simulink model "BDA_DynamicModel_v3"  (R2021b)
settings: Solver=ode23t  StartTime=0.0  StopTime=15  FixedStep=0.000001  MaxStep=1e-5  MinStep=1e-7  RelTol=1e-3
undefined symbols (not defined in the file or in its folder): X, Y, Z
libraries: sm_lib x47, nesl_utility x7
(part 1 of 5)
settings Model: Creator=Alejandro TeveraRuiz  LastModifiedBy=Alejandro TeveraRuiz

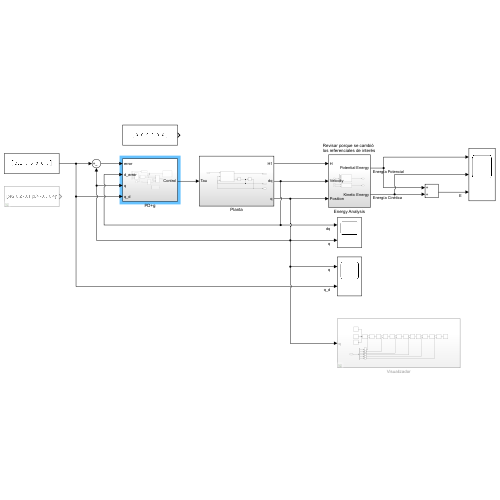
[thumbnail: Simulink's stored preview of the top-level diagram]
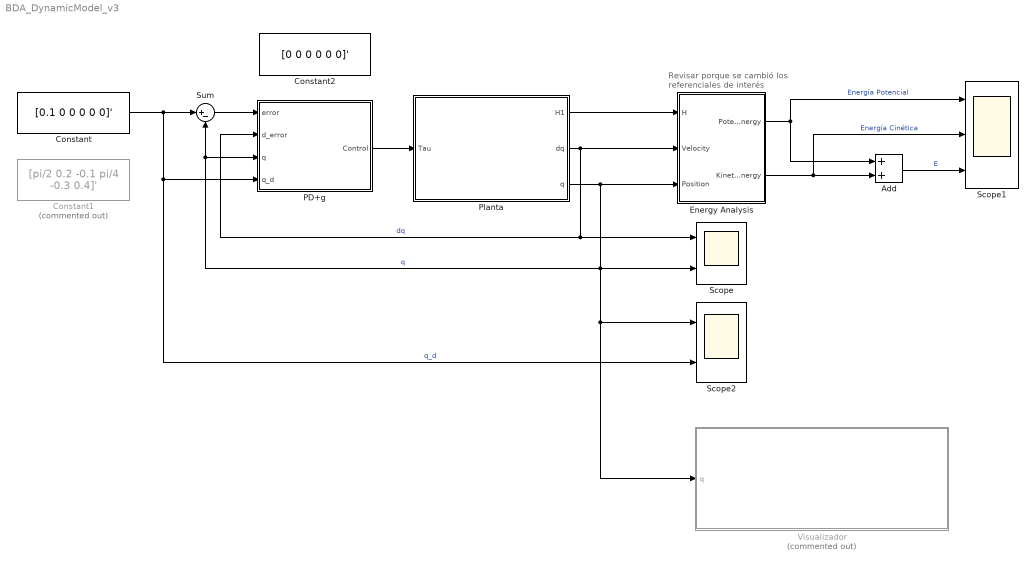
== system BDA_DynamicModel_v3 ==
  note: Revisar porque se cambió los referenciales de interés
  Add : Sum
  Constant : Constant  Value=[0.1 0 0 0 0 0]'
  Constant1 : Constant  Commented=on  Value=[pi/2 0.2 -0.1 pi/4 -0.3 0.4]'
  Constant2 : Constant  Value=[0 0 0 0 0 0]'
  Energy Analysis : Subsystem
  PD+g : Subsystem
  Planta : Subsystem
  Scope : Scope  NumInputPorts=2
  Scope1 : Scope  NumInputPorts=3
  Scope2 : Scope  NumInputPorts=2
  Sum : Sum  Inputs=|+-
  Visualizador : Subsystem  Commented=on
  wires:
  Energy Analysis/1(Potential Energy) -> Scope1/1, Add/1  "Energía Potencial"
  Energy Analysis/2(Kinetic Energy) -> Add/2, Scope1/2  "Energía Cinética"
  Constant/1 -> PD+g/4(q_d), Scope2/2, Sum/1  "q_d"
  Sum/1 -> PD+g/1(error)
  Planta/1(H1) -> Energy Analysis/1(H)
  Planta/2(dq) -> PD+g/2(d_error), Scope/1, Energy Analysis/2(Velocity)  "dq"
  Planta/3(q) -> Energy Analysis/3(Position), Visualizador/1(q), Scope2/1, PD+g/3(q), Sum/2, Scope/2  "q"
  Add/1 -> Scope1/3  "E"
  PD+g/1(Control) -> Planta/1(Tau)

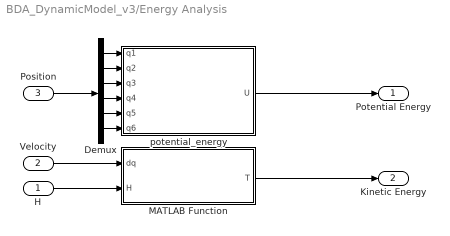
== system BDA_DynamicModel_v3/Energy Analysis ==
  H : Inport
  Velocity : Inport  Port=2
  Position : Inport  Port=3
  Demux : Demux  Outputs=6
  MATLAB Function : MATLAB Function  TreatAsAtomicUnit=on
  potential_energy : MATLAB Function  TreatAsAtomicUnit=on
  Potential Energy : Outport
  Kinetic Energy : Outport  Port=2
  wires:
  Demux/3 -> potential_energy/3(q3)
  Velocity/1 -> MATLAB Function/1(dq)
  Demux/5 -> potential_energy/5(q5)
  Demux/4 -> potential_energy/4(q4)
  Demux/2 -> potential_energy/2(q2)
  Demux/1 -> potential_energy/1(q1)
  Demux/6 -> potential_energy/6(q6)
  H/1 -> MATLAB Function/2(H)
  MATLAB Function/1(T) -> Kinetic Energy/1
  Position/1 -> Demux/1
  potential_energy/1(U) -> Potential Energy/1

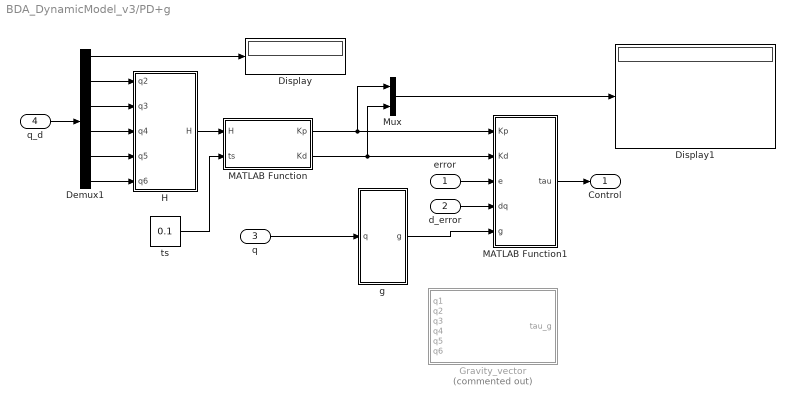
== system BDA_DynamicModel_v3/PD+g ==
  error : Inport
  d_error : Inport  Port=2
  q : Inport  Port=3  PortDimensions=[6,1]
  q_d : Inport  Port=4
  Demux1 : Demux  Outputs=6
  Display : Display
  Display1 : Display
  Gravity_vector : MATLAB Function  Commented=on  TreatAsAtomicUnit=on
  H : MATLAB Function  TreatAsAtomicUnit=on
  MATLAB Function : MATLAB Function  TreatAsAtomicUnit=on
  MATLAB Function1 : MATLAB Function  TreatAsAtomicUnit=on
  Mux : Mux  Inputs=2
  g : MATLAB Function  TreatAsAtomicUnit=on
  ts : Constant  Value=0.1
  Control : Outport
  wires:
  q/1 -> g/1(q)
  g/1(g) -> MATLAB Function1/5(g)
  Demux1/6 -> H/5(q6)
  Demux1/4 -> H/3(q4)
  Demux1/5 -> H/4(q5)
  Demux1/2 -> H/1(q2)
  Demux1/3 -> H/2(q3)
  q_d/1 -> Demux1/1
  H/1(H) -> MATLAB Function/1(H)
  ts/1 -> MATLAB Function/2(ts)
  Demux1/1 -> Display/1
  MATLAB Function/1(Kp) -> Mux/1, MATLAB Function1/1(Kp)
  MATLAB Function/2(Kd) -> Mux/2, MATLAB Function1/2(Kd)
  error/1 -> MATLAB Function1/3(e)
  d_error/1 -> MATLAB Function1/4(dq)
  MATLAB Function1/1(tau) -> Control/1
  Mux/1 -> Display1/1

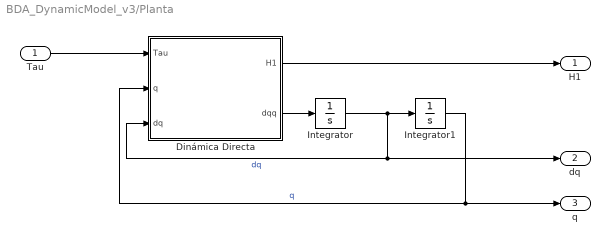
== system BDA_DynamicModel_v3/Planta ==
  Tau : Inport
  Dinámica Directa : Subsystem
  Integrator : Integrator
  Integrator1 : Integrator
  H1 : Outport
  dq : Outport  Port=2
  q : Outport  Port=3
  wires:
  Integrator/1 -> Dinámica Directa/3(dq), dq/1, Integrator1/1  "dq"
  Dinámica Directa/2(dqq) -> Integrator/1
  Integrator1/1 -> Dinámica Directa/2(q), q/1  "q"
  Tau/1 -> Dinámica Directa/1(Tau)
  Dinámica Directa/1(H1) -> H1/1

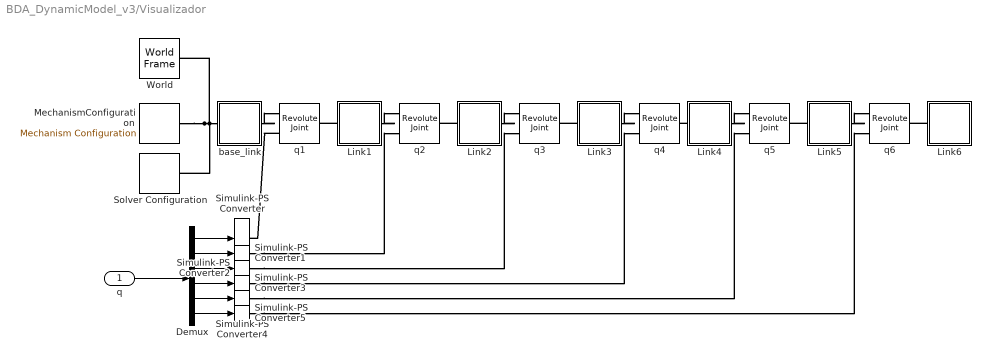
== system BDA_DynamicModel_v3/Visualizador ==
  q : Inport
  Demux : Demux  Outputs=6
  Link1 : Subsystem
  Link2 : Subsystem
  Link3 : Subsystem
  Link4 : Subsystem
  Link5 : Subsystem
  Link6 : Subsystem
  MechanismConfiguration : sm_lib/Utilities/Mechanism Configuration  UniformGravity=None  GravityVector=[0 0 -9.80665]  GravityUnits=m/s^2  LinearizationDelta=0.001  JointModeTransitionNonlinearIterations=2
  Simulink-PS Converter{,1..4} (5 alike) : nesl_utility/Simulink-PS Converter  PhysicalDomain=network_engine_domain  SubClassName=ps_input  LeftPortType=input  RightPortType=output  PseudoPeriodic=off  Frequencies=[]  NoiseDistribution=none  NoiseParameters=[]  Unit=rad  AffineConversion=off  FilteringAndDerivatives=filter  SimscapeFilterOrder=2  InputFilterTimeConstant=0.001  UdotUserProvided=0
      settings: SourceProductBaseCode=PW,SS
  Simulink-PS Converter5 : nesl_utility/Simulink-PS Converter  PhysicalDomain=network_engine_domain  SubClassName=ps_input  LeftPortType=input  RightPortType=output  PseudoPeriodic=off  Frequencies=[]  NoiseDistribution=none  NoiseParameters=[]  Unit=rad  AffineConversion=off  FilteringAndDerivatives=filter  SimscapeFilterOrder=2  InputFilterTimeConstant=0.001  UdotUserProvided=1
      settings: SourceProductBaseCode=PW,SS
  Solver Configuration : nesl_utility/Solver Configuration  PhysicalDomain=network_engine_domain  SubClassName=solver  LeftPortType=input  RightPortType=generic  Tones=[]  Harmonics=[]  SimulateNoise=off  Profile=off  UseLocalSampling=off  EnableSwitchedLinearOptims=on  FrequencyDomain=off  UseCCode=off  RelTol=0.001  AbsTol=1e-06  MinStep=1e-09  ToWorkspace=off  RevertToSquareIcSolve=off  NumHomotopyIterations=100  PhasorMode=off  PhasorModeNumHarmonics=1  DoDC=off  ResidualTolerance=1e-09  UseLocalSolver=off  LocalSolverChoice=NE_BACKWARD_EULER_ADVANCER  LocalSolverSampleTime=0.001  DoFixedCost=off  MaxNonlinIter=3  MaxModeIter=2  ComputeImpulses=off  ImpulseIterations=2  LinearAlgebra=auto  EquationFormulation=NE_TIME_EF  DelaysMemoryBudget=1024  AutomaticFiltering=on  FilteringTimeConstant=0.001  PartitionStorageMethod=AS_NEEDED  PartitionMemoryBudget=1024  PartitionMethod=ROBUST
      settings: SourceProductBaseCode=PW,SS
  World : sm_lib/Frames and Transforms/World Frame
  base_link : Subsystem
  q{1..6} (6 alike) : sm_lib/Joints/Revolute Joint  JointMode=Normal  SenseConstraintForce=off  SenseConstraintForceX=off  SenseConstraintForceY=off  SenseConstraintForceZ=off  SenseConstraintTorque=off  SenseConstraintTorqueX=off  SenseConstraintTorqueY=off  SenseConstraintTorqueZ=off  SenseTotalForce=off  SenseTotalForceX=off  SenseTotalForceY=off  SenseTotalForceZ=off  SenseTotalTorque=off  SenseTotalTorqueX=off  SenseTotalTorqueY=off  SenseTotalTorqueZ=off  CompositeWrenchDir=FollowerOnBase  CompositeWrenchFrame=BaseFrame  EquilibriumPosition=0  EquilibriumPositionUnits=rad  SpringStiffness=0  SpringStiffnessUnits=N*m/deg  DampingCoefficient=0  DampingCoefficientUnits=kg*m^2/(rad*s)  TorqueActuationMode=ComputedTorque  MotionActuationMode=InputMotion  SensePosition=off  SenseVelocity=off  SenseAcceleration=off  SenseTorqueForce=off  SenseLowerLimitTorqueForce=off  SenseUpperLimitTorqueForce=off  LowerLimitSpecify=off  LowerLimitBound=0  LowerLimitBoundUnits=rad  LowerLimitStiffness=1e4  LowerLimitStiffnessUnits=N*m/deg  LowerLimitDamping=10  LowerLimitDampingUnits=N*m/(deg/s)  LowerLimitTransitionRegionWidth=0.1  LowerLimitTransitionRegionWidthUnits=deg  UpperLimitSpecify=off  UpperLimitBound=0  UpperLimitBoundUnits=rad  UpperLimitStiffness=1e4  UpperLimitStiffnessUnits=N*m/deg  UpperLimitDamping=10  UpperLimitDampingUnits=N*m/(deg/s)  UpperLimitTransitionRegionWidth=0.1  UpperLimitTransitionRegionWidthUnits=deg  PositionTargetSpecify=off  PositionTargetPriority=High  PositionTargetValue=0  PositionTargetValueUnits=deg  VelocityTargetSpecify=off  VelocityTargetPriority=High  VelocityTargetValue=0  VelocityTargetValueUnits=deg/s
  wires:
  Demux/6 -> Simulink-PS Converter5/1
  Demux/4 -> Simulink-PS Converter3/1
  Demux/3 -> Simulink-PS Converter2/1
  Demux/1 -> Simulink-PS Converter/1
  Demux/2 -> Simulink-PS Converter1/1
  Demux/5 -> Simulink-PS Converter4/1
  q/1 -> Demux/1
  connections:
  Link3/LConn1 -- q3/RConn1
  Link4/LConn1 -- q4/RConn1
  Simulink-PS Converter3/RConn1 -- q4/LConn2
  Link2/LConn1 -- q2/RConn1
  Simulink-PS Converter4/RConn1 -- q5/LConn2
  base_link/LConn1 -- World/RConn1 -- Solver Configuration/RConn1 -- MechanismConfiguration/RConn1
  Simulink-PS Converter1/RConn1 -- q2/LConn2
  Simulink-PS Converter2/RConn1 -- q3/LConn2
  Link1/RConn1 -- q2/LConn1
  Link2/RConn1 -- q3/LConn1
  q1/LConn2 -- Simulink-PS Converter/RConn1
  Link5/RConn1 -- q6/LConn1
  Link1/LConn1 -- q1/RConn1
  Link3/RConn1 -- q4/LConn1
  Link4/RConn1 -- q5/LConn1
  Simulink-PS Converter5/RConn1 -- q6/LConn2
  Link5/LConn1 -- q5/RConn1
  Link6/LConn1 -- q6/RConn1
  base_link/RConn1 -- q1/LConn1

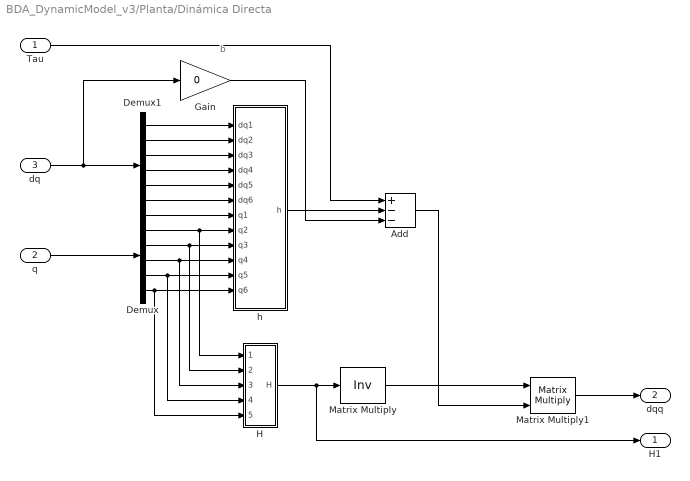
== system BDA_DynamicModel_v3/Planta/Dinámica Directa ==
  note: b
  Tau : Inport
  q : Inport  Port=2
  dq : Inport  Port=3
  Add : Sum  Inputs=+--
  Demux : Demux  Outputs=6
  Demux1 : Demux  Outputs=6
  Gain : Gain  Gain=0
  H : MATLAB Function  TreatAsAtomicUnit=on
  Matrix Multiply : Product  Inputs=/  Multiplication=Matrix(*)
  Matrix Multiply1 : Product  Multiplication=Matrix(*)
  h : MATLAB Function  TreatAsAtomicUnit=on
  H1 : Outport
  dqq : Outport  Port=2
  wires:
  Demux/5 -> H/4(q5), h/11(q5)
  Demux/3 -> H/2(q3), h/9(q3)
  Demux/2 -> H/1(q2), h/8(q2)
  H/1(H) -> H1/1, Matrix Multiply/1
  dq/1 -> Demux1/1, Gain/1
  Gain/1 -> Add/3
  Demux/6 -> H/5(q6), h/12(q6)
  Demux/4 -> H/3(q4), h/10(q4)
  q/1 -> Demux/1
  Matrix Multiply/1 -> Matrix Multiply1/1
  Matrix Multiply1/1 -> dqq/1
  Add/1 -> Matrix Multiply1/2
  Demux1/1 -> h/1(dq1)
  Demux1/2 -> h/2(dq2)
  Demux1/6 -> h/6(dq6)
  Demux/1 -> h/7(q1)
  Demux1/3 -> h/3(dq3)
  Demux1/4 -> h/4(dq4)
  Demux1/5 -> h/5(dq5)
  Tau/1 -> Add/1
  h/1(h) -> Add/2

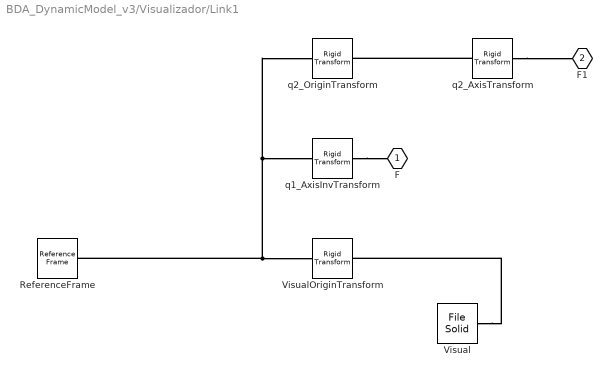
== system BDA_DynamicModel_v3/Visualizador/Link1 ==
  ReferenceFrame : sm_lib/Frames and Transforms/Reference Frame
  Visual : sm_lib/Body Elements/File Solid  ExtGeomFileName=mechanic_model_urdf/meshes/Link1.STL  UnitType=Custom  ExtGeomFileUnits=m  StepReaderType=HEX  ExportConvexHullGeometry=off  InertiaType=PointMass  Mass=1  MassUnits=kg  CenterOfMass=[0, 0, 0]  CenterOfMassUnits=m  MomentsOfInertia=[0, 0, 0]  MomentsOfInertiaUnits=kg*m^2  ProductsOfInertia=[0, 0, 0]  ProductsOfInertiaUnits=kg*m^2  BasedOnType=DensityFromFile  Density=1000  DensityUnits=kg/m^3  DoExposeReferenceFrame=on  SerializedFrames=<Frames/>  GraphicType=FromGeometry  MarkerShape=Sphere  MarkerSize=10  GraphicVisPropType=SimpleVisualProperties  GraphicDiffuseColor=[1.0 1.0 1.0]  GraphicSpecularColor=[0.5 0.5 0.5 1.0]  GraphicAmbientColor=[0.15 0.15 0.15 1.0]  GraphicEmissiveColor=[0.0 0.0 0.0 1.0]  GraphicShininess=75  GraphicOpacity=1
  VisualOriginTransform : sm_lib/Frames and Transforms/Rigid Transform  TranslationMethod=Cartesian  TranslationStandardOffset=0  TranslationLengthUnit=m  TranslationStandardAxis=+Z  TranslationCartesianOffset=[0, 0, 0]  TranslationROffset=0  TranslationROffsetUnits=m  TranslationZOffset=0  TranslationZOffsetUnits=m  TranslationThetaOffset=0  TranslationThetaOffsetUnits=deg  RotationMethod=RotationSequence  RotationAngleUnits=deg  RotationStandardAxis=+Z  RotationAngle=0.0  RotationArbitraryAxis=[0 0 1]  FollAlignAxisA=+X  BaseAlignAxisA=+Y  FollAlignAxisB=+Y  BaseAlignAxisB=+Z  RotationSequenceAxes=BaseAxes  RotationSequence=XYZ  RotationSequenceAngles=[0, 0, 0]  RotationSequenceAnglesUnits=rad  RotationMatrix=[1 0 0; 0 1 0; 0 0 1]
  q1_AxisInvTransform : sm_lib/Frames and Transforms/Rigid Transform  TranslationMethod=Cartesian  TranslationStandardOffset=0  TranslationLengthUnit=m  TranslationStandardAxis=+Z  TranslationCartesianOffset=[0, 0, 0]  TranslationROffset=0  TranslationROffsetUnits=m  TranslationZOffset=0  TranslationZOffsetUnits=m  TranslationThetaOffset=0  TranslationThetaOffsetUnits=deg  RotationMethod=ArbitraryAxis  RotationAngleUnits=rad  RotationStandardAxis=+Z  RotationAngle=1.570796326794897  RotationArbitraryAxis=[-1, 0, 0]  FollAlignAxisA=+X  BaseAlignAxisA=+Y  FollAlignAxisB=+Y  BaseAlignAxisB=+Z  RotationSequenceAxes=FollowerAxes  RotationSequence=XYX  RotationSequenceAngles=[0 0 0]  RotationSequenceAnglesUnits=deg  RotationMatrix=[1 0 0; 0 1 0; 0 0 1]
  q2_AxisTransform : sm_lib/Frames and Transforms/Rigid Transform  TranslationMethod=Cartesian  TranslationStandardOffset=0  TranslationLengthUnit=m  TranslationStandardAxis=+Z  TranslationCartesianOffset=[0, 0, 0]  TranslationROffset=0  TranslationROffsetUnits=m  TranslationZOffset=0  TranslationZOffsetUnits=m  TranslationThetaOffset=0  TranslationThetaOffsetUnits=deg  RotationMethod=ArbitraryAxis  RotationAngleUnits=rad  RotationStandardAxis=+Z  RotationAngle=1.570796326794897  RotationArbitraryAxis=[-1, 0, 0]  FollAlignAxisA=+X  BaseAlignAxisA=+Y  FollAlignAxisB=+Y  BaseAlignAxisB=+Z  RotationSequenceAxes=FollowerAxes  RotationSequence=XYX  RotationSequenceAngles=[0 0 0]  RotationSequenceAnglesUnits=deg  RotationMatrix=[1 0 0; 0 1 0; 0 0 1]
  q2_OriginTransform : sm_lib/Frames and Transforms/Rigid Transform  TranslationMethod=Cartesian  TranslationStandardOffset=0  TranslationLengthUnit=m  TranslationStandardAxis=+Z  TranslationCartesianOffset=[0.032355, 0, 0.10513]  TranslationROffset=0  TranslationROffsetUnits=m  TranslationZOffset=0  TranslationZOffsetUnits=m  TranslationThetaOffset=0  TranslationThetaOffsetUnits=deg  RotationMethod=RotationSequence  RotationAngleUnits=deg  RotationStandardAxis=+Z  RotationAngle=0.0  RotationArbitraryAxis=[0 0 1]  FollAlignAxisA=+X  BaseAlignAxisA=+Y  FollAlignAxisB=+Y  BaseAlignAxisB=+Z  RotationSequenceAxes=BaseAxes  RotationSequence=XYZ  RotationSequenceAngles=[0, 0, 0]  RotationSequenceAnglesUnits=rad  RotationMatrix=[1 0 0; 0 1 0; 0 0 1]
  F : PMIOPort  Side=Left
  F1 : PMIOPort  Port=2  Side=Right
  connections:
  ReferenceFrame/RConn1 -- q1_AxisInvTransform/LConn1 -- q2_OriginTransform/LConn1 -- VisualOriginTransform/LConn1
  Visual/RConn1 -- VisualOriginTransform/RConn1
  q1_AxisInvTransform/RConn1 -- F/RConn1
  q2_AxisTransform/RConn1 -- F1/RConn1
  q2_AxisTransform/LConn1 -- q2_OriginTransform/RConn1

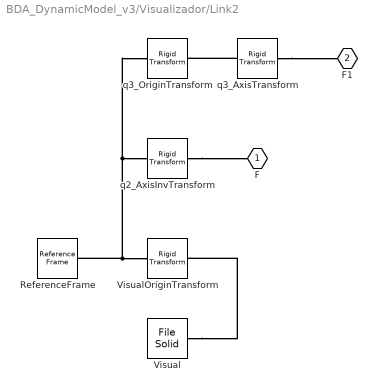
== system BDA_DynamicModel_v3/Visualizador/Link2 ==
  ReferenceFrame : sm_lib/Frames and Transforms/Reference Frame
  Visual : sm_lib/Body Elements/File Solid  ExtGeomFileName=mechanic_model_urdf/meshes/Link2.STL  UnitType=Custom  ExtGeomFileUnits=m  StepReaderType=HEX  ExportConvexHullGeometry=off  InertiaType=PointMass  Mass=0  MassUnits=kg  CenterOfMass=[0, 0, 0]  CenterOfMassUnits=m  MomentsOfInertia=[0, 0, 0]  MomentsOfInertiaUnits=kg*m^2  ProductsOfInertia=[0, 0, 0]  ProductsOfInertiaUnits=kg*m^2  BasedOnType=DensityFromFile  Density=1000  DensityUnits=kg/m^3  DoExposeReferenceFrame=on  SerializedFrames=<Frames/>  GraphicType=FromGeometry  MarkerShape=Sphere  MarkerSize=10  GraphicVisPropType=SimpleVisualProperties  GraphicDiffuseColor=[1.0 1.0 1.0]  GraphicSpecularColor=[0.5 0.5 0.5 1.0]  GraphicAmbientColor=[0.15 0.15 0.15 1.0]  GraphicEmissiveColor=[0.0 0.0 0.0 1.0]  GraphicShininess=75  GraphicOpacity=1
  VisualOriginTransform : sm_lib/Frames and Transforms/Rigid Transform  TranslationMethod=Cartesian  TranslationStandardOffset=0  TranslationLengthUnit=m  TranslationStandardAxis=+Z  TranslationCartesianOffset=[0, 0, 0]  TranslationROffset=0  TranslationROffsetUnits=m  TranslationZOffset=0  TranslationZOffsetUnits=m  TranslationThetaOffset=0  TranslationThetaOffsetUnits=deg  RotationMethod=RotationSequence  RotationAngleUnits=deg  RotationStandardAxis=+Z  RotationAngle=0.0  RotationArbitraryAxis=[0 0 1]  FollAlignAxisA=+X  BaseAlignAxisA=+Y  FollAlignAxisB=+Y  BaseAlignAxisB=+Z  RotationSequenceAxes=BaseAxes  RotationSequence=XYZ  RotationSequenceAngles=[0, 0, 0]  RotationSequenceAnglesUnits=rad  RotationMatrix=[1 0 0; 0 1 0; 0 0 1]
  q2_AxisInvTransform : sm_lib/Frames and Transforms/Rigid Transform  TranslationMethod=Cartesian  TranslationStandardOffset=0  TranslationLengthUnit=m  TranslationStandardAxis=+Z  TranslationCartesianOffset=[0, 0, 0]  TranslationROffset=0  TranslationROffsetUnits=m  TranslationZOffset=0  TranslationZOffsetUnits=m  TranslationThetaOffset=0  TranslationThetaOffsetUnits=deg  RotationMethod=ArbitraryAxis  RotationAngleUnits=rad  RotationStandardAxis=+Z  RotationAngle=1.570796326794897  RotationArbitraryAxis=[-1, 0, 0]  FollAlignAxisA=+X  BaseAlignAxisA=+Y  FollAlignAxisB=+Y  BaseAlignAxisB=+Z  RotationSequenceAxes=FollowerAxes  RotationSequence=XYX  RotationSequenceAngles=[0 0 0]  RotationSequenceAnglesUnits=deg  RotationMatrix=[1 0 0; 0 1 0; 0 0 1]
  q3_AxisTransform : sm_lib/Frames and Transforms/Rigid Transform  TranslationMethod=Cartesian  TranslationStandardOffset=0  TranslationLengthUnit=m  TranslationStandardAxis=+Z  TranslationCartesianOffset=[0, 0, 0]  TranslationROffset=0  TranslationROffsetUnits=m  TranslationZOffset=0  TranslationZOffsetUnits=m  TranslationThetaOffset=0  TranslationThetaOffsetUnits=deg  RotationMethod=ArbitraryAxis  RotationAngleUnits=rad  RotationStandardAxis=+Z  RotationAngle=0.9820504269198674  RotationArbitraryAxis=[-0, -0.831637757907627, 0]  FollAlignAxisA=+X  BaseAlignAxisA=+Y  FollAlignAxisB=+Y  BaseAlignAxisB=+Z  RotationSequenceAxes=FollowerAxes  RotationSequence=XYX  RotationSequenceAngles=[0 0 0]  RotationSequenceAnglesUnits=deg  RotationMatrix=[1 0 0; 0 1 0; 0 0 1]
  q3_OriginTransform : sm_lib/Frames and Transforms/Rigid Transform  TranslationMethod=Cartesian  TranslationStandardOffset=0  TranslationLengthUnit=m  TranslationStandardAxis=+Z  TranslationCartesianOffset=[-0.036138, 0, 0.025038]  TranslationROffset=0  TranslationROffsetUnits=m  TranslationZOffset=0  TranslationZOffsetUnits=m  TranslationThetaOffset=0  TranslationThetaOffsetUnits=deg  RotationMethod=RotationSequence  RotationAngleUnits=deg  RotationStandardAxis=+Z  RotationAngle=0.0  RotationArbitraryAxis=[0 0 1]  FollAlignAxisA=+X  BaseAlignAxisA=+Y  FollAlignAxisB=+Y  BaseAlignAxisB=+Z  RotationSequenceAxes=BaseAxes  RotationSequence=XYZ  RotationSequenceAngles=[0, 0, 0]  RotationSequenceAnglesUnits=rad  RotationMatrix=[1 0 0; 0 1 0; 0 0 1]
  F : PMIOPort  Side=Left
  F1 : PMIOPort  Port=2  Side=Right
  connections:
  ReferenceFrame/RConn1 -- q2_AxisInvTransform/LConn1 -- q3_OriginTransform/LConn1 -- VisualOriginTransform/LConn1
  Visual/RConn1 -- VisualOriginTransform/RConn1
  q2_AxisInvTransform/RConn1 -- F/RConn1
  q3_AxisTransform/RConn1 -- F1/RConn1
  q3_AxisTransform/LConn1 -- q3_OriginTransform/RConn1

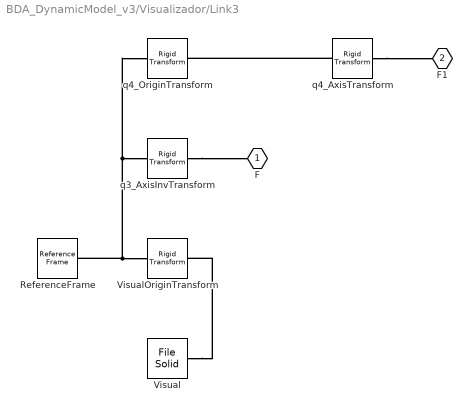
== system BDA_DynamicModel_v3/Visualizador/Link3 ==
  ReferenceFrame : sm_lib/Frames and Transforms/Reference Frame
  Visual : sm_lib/Body Elements/File Solid  ExtGeomFileName=mechanic_model_urdf/meshes/Link3.STL  UnitType=Custom  ExtGeomFileUnits=m  StepReaderType=HEX  ExportConvexHullGeometry=off  InertiaType=PointMass  Mass=0  MassUnits=kg  CenterOfMass=[0, 0, 0]  CenterOfMassUnits=m  MomentsOfInertia=[0, 0, 0]  MomentsOfInertiaUnits=kg*m^2  ProductsOfInertia=[0, 0, 0]  ProductsOfInertiaUnits=kg*m^2  BasedOnType=DensityFromFile  Density=1000  DensityUnits=kg/m^3  DoExposeReferenceFrame=on  SerializedFrames=<Frames/>  GraphicType=FromGeometry  MarkerShape=Sphere  MarkerSize=10  GraphicVisPropType=SimpleVisualProperties  GraphicDiffuseColor=[1, 1, 1]  GraphicSpecularColor=[0.5 0.5 0.5 1.0]  GraphicAmbientColor=[0.15 0.15 0.15 1.0]  GraphicEmissiveColor=[0.0 0.0 0.0 1.0]  GraphicShininess=75  GraphicOpacity=1
  VisualOriginTransform : sm_lib/Frames and Transforms/Rigid Transform  TranslationMethod=Cartesian  TranslationStandardOffset=0  TranslationLengthUnit=m  TranslationStandardAxis=+Z  TranslationCartesianOffset=[0, 0, 0]  TranslationROffset=0  TranslationROffsetUnits=m  TranslationZOffset=0  TranslationZOffsetUnits=m  TranslationThetaOffset=0  TranslationThetaOffsetUnits=deg  RotationMethod=RotationSequence  RotationAngleUnits=deg  RotationStandardAxis=+Z  RotationAngle=0.0  RotationArbitraryAxis=[0 0 1]  FollAlignAxisA=+X  BaseAlignAxisA=+Y  FollAlignAxisB=+Y  BaseAlignAxisB=+Z  RotationSequenceAxes=BaseAxes  RotationSequence=XYZ  RotationSequenceAngles=[0, 0, 0]  RotationSequenceAnglesUnits=rad  RotationMatrix=[1 0 0; 0 1 0; 0 0 1]
  q3_AxisInvTransform : sm_lib/Frames and Transforms/Rigid Transform  TranslationMethod=Cartesian  TranslationStandardOffset=0  TranslationLengthUnit=m  TranslationStandardAxis=+Z  TranslationCartesianOffset=[0, 0, 0]  TranslationROffset=0  TranslationROffsetUnits=m  TranslationZOffset=0  TranslationZOffsetUnits=m  TranslationThetaOffset=0  TranslationThetaOffsetUnits=deg  RotationMethod=ArbitraryAxis  RotationAngleUnits=rad  RotationStandardAxis=+Z  RotationAngle=0.9820504269198674  RotationArbitraryAxis=[-0, -0.831637757907627, 0]  FollAlignAxisA=+X  BaseAlignAxisA=+Y  FollAlignAxisB=+Y  BaseAlignAxisB=+Z  RotationSequenceAxes=FollowerAxes  RotationSequence=XYX  RotationSequenceAngles=[0 0 0]  RotationSequenceAnglesUnits=deg  RotationMatrix=[1 0 0; 0 1 0; 0 0 1]
  q4_AxisTransform : sm_lib/Frames and Transforms/Rigid Transform  TranslationMethod=Cartesian  TranslationStandardOffset=0  TranslationLengthUnit=m  TranslationStandardAxis=+Z  TranslationCartesianOffset=[0, 0, 0]  TranslationROffset=0  TranslationROffsetUnits=m  TranslationZOffset=0  TranslationZOffsetUnits=m  TranslationThetaOffset=0  TranslationThetaOffsetUnits=deg  RotationMethod=ArbitraryAxis  RotationAngleUnits=rad  RotationStandardAxis=+Z  RotationAngle=0  RotationArbitraryAxis=[1, 0, 0]  FollAlignAxisA=+X  BaseAlignAxisA=+Y  FollAlignAxisB=+Y  BaseAlignAxisB=+Z  RotationSequenceAxes=FollowerAxes  RotationSequence=XYX  RotationSequenceAngles=[0 0 0]  RotationSequenceAnglesUnits=deg  RotationMatrix=[1 0 0; 0 1 0; 0 0 1]
  q4_OriginTransform : sm_lib/Frames and Transforms/Rigid Transform  TranslationMethod=Cartesian  TranslationStandardOffset=0  TranslationLengthUnit=m  TranslationStandardAxis=+Z  TranslationCartesianOffset=[-0.012178, 0, 0.021314]  TranslationROffset=0  TranslationROffsetUnits=m  TranslationZOffset=0  TranslationZOffsetUnits=m  TranslationThetaOffset=0  TranslationThetaOffsetUnits=deg  RotationMethod=RotationSequence  RotationAngleUnits=deg  RotationStandardAxis=+Z  RotationAngle=0.0  RotationArbitraryAxis=[0 0 1]  FollAlignAxisA=+X  BaseAlignAxisA=+Y  FollAlignAxisB=+Y  BaseAlignAxisB=+Z  RotationSequenceAxes=BaseAxes  RotationSequence=XYZ  RotationSequenceAngles=[0, 0, 0]  RotationSequenceAnglesUnits=rad  RotationMatrix=[1 0 0; 0 1 0; 0 0 1]
  F : PMIOPort  Side=Left
  F1 : PMIOPort  Port=2  Side=Right
  connections:
  ReferenceFrame/RConn1 -- q3_AxisInvTransform/LConn1 -- q4_OriginTransform/LConn1 -- VisualOriginTransform/LConn1
  Visual/RConn1 -- VisualOriginTransform/RConn1
  q3_AxisInvTransform/RConn1 -- F/RConn1
  q4_AxisTransform/RConn1 -- F1/RConn1
  q4_AxisTransform/LConn1 -- q4_OriginTransform/RConn1

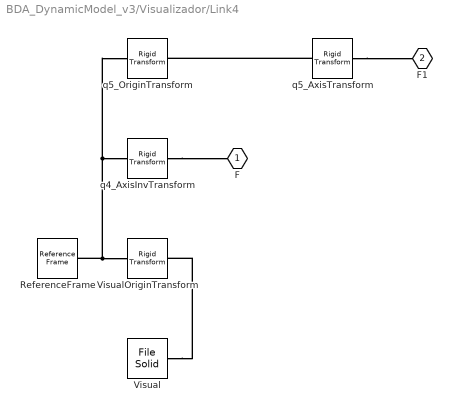
== system BDA_DynamicModel_v3/Visualizador/Link4 ==
  ReferenceFrame : sm_lib/Frames and Transforms/Reference Frame
  Visual : sm_lib/Body Elements/File Solid  ExtGeomFileName=mechanic_model_urdf/meshes/Link4.STL  UnitType=Custom  ExtGeomFileUnits=m  StepReaderType=HEX  ExportConvexHullGeometry=off  InertiaType=PointMass  Mass=0  MassUnits=kg  CenterOfMass=[0, 0, 0]  CenterOfMassUnits=m  MomentsOfInertia=[0, 0, 0]  MomentsOfInertiaUnits=kg*m^2  ProductsOfInertia=[0, 0, 0]  ProductsOfInertiaUnits=kg*m^2  BasedOnType=DensityFromFile  Density=1000  DensityUnits=kg/m^3  DoExposeReferenceFrame=on  SerializedFrames=<Frames/>  GraphicType=FromGeometry  MarkerShape=Sphere  MarkerSize=10  GraphicVisPropType=SimpleVisualProperties  GraphicDiffuseColor=[1.0 1.0 1.0]  GraphicSpecularColor=[0.5 0.5 0.5 1.0]  GraphicAmbientColor=[0.15 0.15 0.15 1.0]  GraphicEmissiveColor=[0.0 0.0 0.0 1.0]  GraphicShininess=75  GraphicOpacity=1
  VisualOriginTransform : sm_lib/Frames and Transforms/Rigid Transform  TranslationMethod=Cartesian  TranslationStandardOffset=0  TranslationLengthUnit=m  TranslationStandardAxis=+Z  TranslationCartesianOffset=[0, 0, 0]  TranslationROffset=0  TranslationROffsetUnits=m  TranslationZOffset=0  TranslationZOffsetUnits=m  TranslationThetaOffset=0  TranslationThetaOffsetUnits=deg  RotationMethod=RotationSequence  RotationAngleUnits=deg  RotationStandardAxis=+Z  RotationAngle=0.0  RotationArbitraryAxis=[0 0 1]  FollAlignAxisA=+X  BaseAlignAxisA=+Y  FollAlignAxisB=+Y  BaseAlignAxisB=+Z  RotationSequenceAxes=BaseAxes  RotationSequence=XYZ  RotationSequenceAngles=[0, 0, 0]  RotationSequenceAnglesUnits=rad  RotationMatrix=[1 0 0; 0 1 0; 0 0 1]
  q4_AxisInvTransform : sm_lib/Frames and Transforms/Rigid Transform  TranslationMethod=Cartesian  TranslationStandardOffset=0  TranslationLengthUnit=m  TranslationStandardAxis=+Z  TranslationCartesianOffset=[0, 0, 0]  TranslationROffset=0  TranslationROffsetUnits=m  TranslationZOffset=0  TranslationZOffsetUnits=m  TranslationThetaOffset=0  TranslationThetaOffsetUnits=deg  RotationMethod=ArbitraryAxis  RotationAngleUnits=rad  RotationStandardAxis=+Z  RotationAngle=0  RotationArbitraryAxis=[1, 0, 0]  FollAlignAxisA=+X  BaseAlignAxisA=+Y  FollAlignAxisB=+Y  BaseAlignAxisB=+Z  RotationSequenceAxes=FollowerAxes  RotationSequence=XYX  RotationSequenceAngles=[0 0 0]  RotationSequenceAnglesUnits=deg  RotationMatrix=[1 0 0; 0 1 0; 0 0 1]
  q5_AxisTransform : sm_lib/Frames and Transforms/Rigid Transform  TranslationMethod=Cartesian  TranslationStandardOffset=0  TranslationLengthUnit=m  TranslationStandardAxis=+Z  TranslationCartesianOffset=[0, 0, 0]  TranslationROffset=0  TranslationROffsetUnits=m  TranslationZOffset=0  TranslationZOffsetUnits=m  TranslationThetaOffset=0  TranslationThetaOffsetUnits=deg  RotationMethod=ArbitraryAxis  RotationAngleUnits=rad  RotationStandardAxis=+Z  RotationAngle=1.570796326794897  RotationArbitraryAxis=[-0, 1, 0]  FollAlignAxisA=+X  BaseAlignAxisA=+Y  FollAlignAxisB=+Y  BaseAlignAxisB=+Z  RotationSequenceAxes=FollowerAxes  RotationSequence=XYX  RotationSequenceAngles=[0 0 0]  RotationSequenceAnglesUnits=deg  RotationMatrix=[1 0 0; 0 1 0; 0 0 1]
  q5_OriginTransform : sm_lib/Frames and Transforms/Rigid Transform  TranslationMethod=Cartesian  TranslationStandardOffset=0  TranslationLengthUnit=m  TranslationStandardAxis=+Z  TranslationCartesianOffset=[-0.00017999, 0, 0.042341]  TranslationROffset=0  TranslationROffsetUnits=m  TranslationZOffset=0  TranslationZOffsetUnits=m  TranslationThetaOffset=0  TranslationThetaOffsetUnits=deg  RotationMethod=RotationSequence  RotationAngleUnits=deg  RotationStandardAxis=+Z  RotationAngle=0.0  RotationArbitraryAxis=[0 0 1]  FollAlignAxisA=+X  BaseAlignAxisA=+Y  FollAlignAxisB=+Y  BaseAlignAxisB=+Z  RotationSequenceAxes=BaseAxes  RotationSequence=XYZ  RotationSequenceAngles=[0, 0, 0]  RotationSequenceAnglesUnits=rad  RotationMatrix=[1 0 0; 0 1 0; 0 0 1]
  F : PMIOPort  Side=Left
  F1 : PMIOPort  Port=2  Side=Right
  connections:
  ReferenceFrame/RConn1 -- q4_AxisInvTransform/LConn1 -- q5_OriginTransform/LConn1 -- VisualOriginTransform/LConn1
  Visual/RConn1 -- VisualOriginTransform/RConn1
  q4_AxisInvTransform/RConn1 -- F/RConn1
  q5_AxisTransform/RConn1 -- F1/RConn1
  q5_AxisTransform/LConn1 -- q5_OriginTransform/RConn1

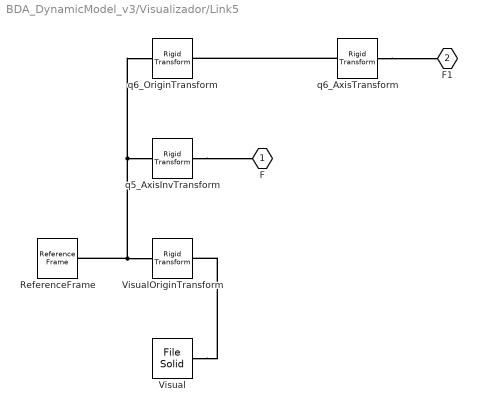
== system BDA_DynamicModel_v3/Visualizador/Link5 ==
  ReferenceFrame : sm_lib/Frames and Transforms/Reference Frame
  Visual : sm_lib/Body Elements/File Solid  ExtGeomFileName=mechanic_model_urdf/meshes/Link5.STL  UnitType=Custom  ExtGeomFileUnits=m  StepReaderType=HEX  ExportConvexHullGeometry=off  InertiaType=PointMass  Mass=0  MassUnits=kg  CenterOfMass=[0, 0, 0]  CenterOfMassUnits=m  MomentsOfInertia=[0, 0, 0]  MomentsOfInertiaUnits=kg*m^2  ProductsOfInertia=[0, 0, 0]  ProductsOfInertiaUnits=kg*m^2  BasedOnType=DensityFromFile  Density=1000  DensityUnits=kg/m^3  DoExposeReferenceFrame=on  SerializedFrames=<Frames/>  GraphicType=FromGeometry  MarkerShape=Sphere  MarkerSize=10  GraphicVisPropType=SimpleVisualProperties  GraphicDiffuseColor=[1.0 1.0 1.0]  GraphicSpecularColor=[0.5 0.5 0.5 1.0]  GraphicAmbientColor=[0.15 0.15 0.15 1.0]  GraphicEmissiveColor=[0.0 0.0 0.0 1.0]  GraphicShininess=75  GraphicOpacity=1
  VisualOriginTransform : sm_lib/Frames and Transforms/Rigid Transform  TranslationMethod=Cartesian  TranslationStandardOffset=0  TranslationLengthUnit=m  TranslationStandardAxis=+Z  TranslationCartesianOffset=[0, 0, 0]  TranslationROffset=0  TranslationROffsetUnits=m  TranslationZOffset=0  TranslationZOffsetUnits=m  TranslationThetaOffset=0  TranslationThetaOffsetUnits=deg  RotationMethod=RotationSequence  RotationAngleUnits=deg  RotationStandardAxis=+Z  RotationAngle=0.0  RotationArbitraryAxis=[0 0 1]  FollAlignAxisA=+X  BaseAlignAxisA=+Y  FollAlignAxisB=+Y  BaseAlignAxisB=+Z  RotationSequenceAxes=BaseAxes  RotationSequence=XYZ  RotationSequenceAngles=[0, 0, 0]  RotationSequenceAnglesUnits=rad  RotationMatrix=[1 0 0; 0 1 0; 0 0 1]
  q5_AxisInvTransform : sm_lib/Frames and Transforms/Rigid Transform  TranslationMethod=Cartesian  TranslationStandardOffset=0  TranslationLengthUnit=m  TranslationStandardAxis=+Z  TranslationCartesianOffset=[0, 0, 0]  TranslationROffset=0  TranslationROffsetUnits=m  TranslationZOffset=0  TranslationZOffsetUnits=m  TranslationThetaOffset=0  TranslationThetaOffsetUnits=deg  RotationMethod=ArbitraryAxis  RotationAngleUnits=rad  RotationStandardAxis=+Z  RotationAngle=1.570796326794897  RotationArbitraryAxis=[-0, 1, 0]  FollAlignAxisA=+X  BaseAlignAxisA=+Y  FollAlignAxisB=+Y  BaseAlignAxisB=+Z  RotationSequenceAxes=FollowerAxes  RotationSequence=XYX  RotationSequenceAngles=[0 0 0]  RotationSequenceAnglesUnits=deg  RotationMatrix=[1 0 0; 0 1 0; 0 0 1]
  q6_AxisTransform : sm_lib/Frames and Transforms/Rigid Transform  TranslationMethod=Cartesian  TranslationStandardOffset=0  TranslationLengthUnit=m  TranslationStandardAxis=+Z  TranslationCartesianOffset=[0, 0, 0]  TranslationROffset=0  TranslationROffsetUnits=m  TranslationZOffset=0  TranslationZOffsetUnits=m  TranslationThetaOffset=0  TranslationThetaOffsetUnits=deg  RotationMethod=ArbitraryAxis  RotationAngleUnits=rad  RotationStandardAxis=+Z  RotationAngle=1.570796326794897  RotationArbitraryAxis=[-1, 0, 0]  FollAlignAxisA=+X  BaseAlignAxisA=+Y  FollAlignAxisB=+Y  BaseAlignAxisB=+Z  RotationSequenceAxes=FollowerAxes  RotationSequence=XYX  RotationSequenceAngles=[0 0 0]  RotationSequenceAnglesUnits=deg  RotationMatrix=[1 0 0; 0 1 0; 0 0 1]
  q6_OriginTransform : sm_lib/Frames and Transforms/Rigid Transform  TranslationMethod=Cartesian  TranslationStandardOffset=0  TranslationLengthUnit=m  TranslationStandardAxis=+Z  TranslationCartesianOffset=[0, 0, 0.006]  TranslationROffset=0  TranslationROffsetUnits=m  TranslationZOffset=0  TranslationZOffsetUnits=m  TranslationThetaOffset=0  TranslationThetaOffsetUnits=deg  RotationMethod=RotationSequence  RotationAngleUnits=deg  RotationStandardAxis=+Z  RotationAngle=0.0  RotationArbitraryAxis=[0 0 1]  FollAlignAxisA=+X  BaseAlignAxisA=+Y  FollAlignAxisB=+Y  BaseAlignAxisB=+Z  RotationSequenceAxes=BaseAxes  RotationSequence=XYZ  RotationSequenceAngles=[0, 0, 0]  RotationSequenceAnglesUnits=rad  RotationMatrix=[1 0 0; 0 1 0; 0 0 1]
  F : PMIOPort  Side=Left
  F1 : PMIOPort  Port=2  Side=Right
  connections:
  ReferenceFrame/RConn1 -- q5_AxisInvTransform/LConn1 -- q6_OriginTransform/LConn1 -- VisualOriginTransform/LConn1
  Visual/RConn1 -- VisualOriginTransform/RConn1
  q5_AxisInvTransform/RConn1 -- F/RConn1
  q6_AxisTransform/RConn1 -- F1/RConn1
  q6_AxisTransform/LConn1 -- q6_OriginTransform/RConn1

== system BDA_DynamicModel_v3/Visualizador/Link6 ==
  ReferenceFrame : sm_lib/Frames and Transforms/Reference Frame
  Visual : sm_lib/Body Elements/File Solid  ExtGeomFileName=mechanic_model_urdf/meshes/Link6.STL  UnitType=Custom  ExtGeomFileUnits=m  StepReaderType=HEX  ExportConvexHullGeometry=off  InertiaType=PointMass  Mass=0  MassUnits=kg  CenterOfMass=[0, 0, 0]  CenterOfMassUnits=m  MomentsOfInertia=[0, 0, 0]  MomentsOfInertiaUnits=kg*m^2  ProductsOfInertia=[0, 0, 0]  ProductsOfInertiaUnits=kg*m^2  BasedOnType=DensityFromFile  Density=1000  DensityUnits=kg/m^3  DoExposeReferenceFrame=on  SerializedFrames=<Frames/>  GraphicType=FromGeometry  MarkerShape=Sphere  MarkerSize=10  GraphicVisPropType=SimpleVisualProperties  GraphicDiffuseColor=[1.0 1.0 1.0]  GraphicSpecularColor=[0.5 0.5 0.5 1.0]  GraphicAmbientColor=[0.15 0.15 0.15 1.0]  GraphicEmissiveColor=[0.0 0.0 0.0 1.0]  GraphicShininess=75  GraphicOpacity=0.85
  VisualOriginTransform : sm_lib/Frames and Transforms/Rigid Transform  TranslationMethod=Cartesian  TranslationStandardOffset=0  TranslationLengthUnit=m  TranslationStandardAxis=+Z  TranslationCartesianOffset=[0, 0, 0]  TranslationROffset=0  TranslationROffsetUnits=m  TranslationZOffset=0  TranslationZOffsetUnits=m  TranslationThetaOffset=0  TranslationThetaOffsetUnits=deg  RotationMethod=RotationSequence  RotationAngleUnits=deg  RotationStandardAxis=+Z  RotationAngle=0.0  RotationArbitraryAxis=[0 0 1]  FollAlignAxisA=+X  BaseAlignAxisA=+Y  FollAlignAxisB=+Y  BaseAlignAxisB=+Z  RotationSequenceAxes=BaseAxes  RotationSequence=XYZ  RotationSequenceAngles=[0, 0, 0]  RotationSequenceAnglesUnits=rad  RotationMatrix=[1 0 0; 0 1 0; 0 0 1]
  q6_AxisInvTransform : sm_lib/Frames and Transforms/Rigid Transform  TranslationMethod=Cartesian  TranslationStandardOffset=0  TranslationLengthUnit=m  TranslationStandardAxis=+Z  TranslationCartesianOffset=[0, 0, 0]  TranslationROffset=0  TranslationROffsetUnits=m  TranslationZOffset=0  TranslationZOffsetUnits=m  TranslationThetaOffset=0  TranslationThetaOffsetUnits=deg  RotationMethod=ArbitraryAxis  RotationAngleUnits=rad  RotationStandardAxis=+Z  RotationAngle=1.570796326794897  RotationArbitraryAxis=[-1, 0, 0]  FollAlignAxisA=+X  BaseAlignAxisA=+Y  FollAlignAxisB=+Y  BaseAlignAxisB=+Z  RotationSequenceAxes=FollowerAxes  RotationSequence=XYX  RotationSequenceAngles=[0 0 0]  RotationSequenceAnglesUnits=deg  RotationMatrix=[1 0 0; 0 1 0; 0 0 1]
  F : PMIOPort  Side=Left
  connections:
  ReferenceFrame/RConn1 -- VisualOriginTransform/LConn1 -- q6_AxisInvTransform/LConn1
  Visual/RConn1 -- VisualOriginTransform/RConn1
  q6_AxisInvTransform/RConn1 -- F/RConn1

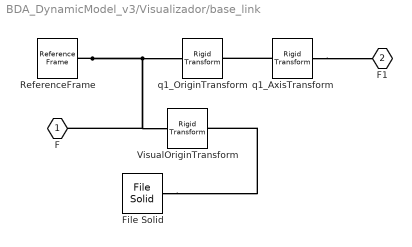
== system BDA_DynamicModel_v3/Visualizador/base_link ==
  File Solid : sm_lib/Body Elements/File Solid  ExtGeomFileName=mechanic_model_urdf\meshes\base_link.STL  UnitType=Custom  ExtGeomFileUnits=m  StepReaderType=HEX  ExportConvexHullGeometry=off  InertiaType=PointMass  Mass=0  MassUnits=kg  CenterOfMass=[0 0 0]  CenterOfMassUnits=m  MomentsOfInertia=[1 1 1]  MomentsOfInertiaUnits=kg*m^2  ProductsOfInertia=[0 0 0]  ProductsOfInertiaUnits=kg*m^2  BasedOnType=DensityFromFile  Density=1000  DensityUnits=kg/m^3  DoExposeReferenceFrame=on  SerializedFrames=<Frames/>  GraphicType=FromGeometry  MarkerShape=Sphere  MarkerSize=10  GraphicVisPropType=SimpleVisualProperties  GraphicDiffuseColor=[1.0 1.0 1.0]  GraphicSpecularColor=[0.5 0.5 0.5 1.0]  GraphicAmbientColor=[0.15 0.15 0.15 1.0]  GraphicEmissiveColor=[0.0 0.0 0.0 1.0]  GraphicShininess=75  GraphicOpacity=1.0
  ReferenceFrame : sm_lib/Frames and Transforms/Reference Frame
  VisualOriginTransform : sm_lib/Frames and Transforms/Rigid Transform  TranslationMethod=Cartesian  TranslationStandardOffset=0  TranslationLengthUnit=cm  TranslationStandardAxis=+Z  TranslationCartesianOffset=[0, 0, 0]  TranslationROffset=0  TranslationROffsetUnits=m  TranslationZOffset=0  TranslationZOffsetUnits=m  TranslationThetaOffset=0  TranslationThetaOffsetUnits=deg  RotationMethod=None  RotationAngleUnits=deg  RotationStandardAxis=+Z  RotationAngle=0.0  RotationArbitraryAxis=[0 0 1]  FollAlignAxisA=+X  BaseAlignAxisA=+Y  FollAlignAxisB=+Y  BaseAlignAxisB=+Z  RotationSequenceAxes=BaseAxes  RotationSequence=XYZ  RotationSequenceAngles=[0, 0, 0]  RotationSequenceAnglesUnits=rad  RotationMatrix=[1 0 0; 0 1 0; 0 0 1]
  q1_AxisTransform : sm_lib/Frames and Transforms/Rigid Transform  TranslationMethod=Cartesian  TranslationStandardOffset=0  TranslationLengthUnit=m  TranslationStandardAxis=+Z  TranslationCartesianOffset=[0, 0, 0]  TranslationROffset=0  TranslationROffsetUnits=m  TranslationZOffset=0  TranslationZOffsetUnits=m  TranslationThetaOffset=0  TranslationThetaOffsetUnits=deg  RotationMethod=ArbitraryAxis  RotationAngleUnits=rad  RotationStandardAxis=+Z  RotationAngle=1.570796326794897  RotationArbitraryAxis=[-1, 0, 0]  FollAlignAxisA=+X  BaseAlignAxisA=+Y  FollAlignAxisB=+Y  BaseAlignAxisB=+Z  RotationSequenceAxes=FollowerAxes  RotationSequence=XYX  RotationSequenceAngles=[0 0 0]  RotationSequenceAnglesUnits=deg  RotationMatrix=[1 0 0; 0 1 0; 0 0 1]
  q1_OriginTransform : sm_lib/Frames and Transforms/Rigid Transform  TranslationMethod=Cartesian  TranslationStandardOffset=0  TranslationLengthUnit=m  TranslationStandardAxis=+Z  TranslationCartesianOffset=[0, 0, 0]  TranslationROffset=0  TranslationROffsetUnits=m  TranslationZOffset=0  TranslationZOffsetUnits=m  TranslationThetaOffset=0  TranslationThetaOffsetUnits=deg  RotationMethod=RotationSequence  RotationAngleUnits=deg  RotationStandardAxis=+Z  RotationAngle=0.0  RotationArbitraryAxis=[0 0 1]  FollAlignAxisA=+X  BaseAlignAxisA=+Y  FollAlignAxisB=+Y  BaseAlignAxisB=+Z  RotationSequenceAxes=BaseAxes  RotationSequence=XYZ  RotationSequenceAngles=[0, 0, 0]  RotationSequenceAnglesUnits=rad  RotationMatrix=[1 0 0; 0 1 0; 0 0 1]
  F : PMIOPort  Side=Left
  F1 : PMIOPort  Port=2  Side=Right
  connections:
  ReferenceFrame/RConn1 -- F/RConn1 -- VisualOriginTransform/LConn1 -- q1_OriginTransform/LConn1
  File Solid/RConn1 -- VisualOriginTransform/RConn1
  q1_AxisTransform/RConn1 -- F1/RConn1
  q1_AxisTransform/LConn1 -- q1_OriginTransform/RConn1

== matlab function BDA_DynamicModel_v3/PD+g/g ==
  data: q input; g output
function g = g(q)
%#codegen
q1 = q(1);
q2 = q(2);
q3 = q(3);
q4 = q(4);
q5 = q(5);
q6 = q(6);
%    This function was generated by the Symbolic Math Toolbox version 9.0.
%    28-Nov-2021 14:48:27

t2 = cos(q2);
t3 = cos(q4);
t4 = cos(q5);
t5 = cos(q6);
t6 = sin(q2);
t7 = sin(q4);
t8 = sin(q5);
t9 = sin(q6);
t15 = 9.007199254740992e+15;
t10 = t2.*1.051339e-1;
t11 = t6.*1.051339e-1;
t13 = t8.*5.110348748545983e-1;
t14 = t6.*3.235525e-2;
t16 = t2.*3.235525e-2;
t17 = t4.*t7.*8.595599785252598e-1;
t18 = (q3.*t15)./9.007199254740992e+15;
t21 = q3.*t15.*1.110223024625157e-16i;
t12 = -t11;
t19 = cos(t18);
t20 = sin(t18);
t22 = exp(t21);
t23 = -t21;
t29 = t10+t14;
t31 = t13+t17;
t24 = 1.0./t22;
t25 = t3.*t19;
t26 = t7.*t19;
t27 = t22-1.0;
t30 = t12+t16;
t32 = t19.*1.273194e-2;
t35 = t19.*3.42298471896e-5;
t36 = t19.*3.07913148585e-5;
t37 = t22.*3.694216783411725e-1;
t38 = t22.*1.305783216588275e-1;
t42 = t19.*3.609174932280216e-3;
t47 = t3.*t15.*t20.*5.673626844500105e-17;
t48 = t7.*t15.*t20.*5.673626844500105e-17;
t49 = t8.*t15.*t20.*9.543032792050485e-17;
t51 = t22.*3.215186923359161e-3;
t53 = t22.*1.345257168956303e-2;
t55 = t15.*t20.*4.87211480085e-18;
t56 = t3.*t15.*t20.*2.479366200131245e-18;
t57 = t3.*t15.*t20.*7.351481000981246e-18;
t58 = t7.*t15.*t20.*9.810473427588925e-18;
t59 = t7.*t15.*t20.*4.938358626738924e-18;
t62 = t22.*1.073174736839591e-5;
t63 = t22.*4.490239736257417e-5;
t66 = t22.*3.813455334903668e-3;
t70 = t8.*t15.*t20.*6.931587185740596e-21;
t71 = t3.*t15.*t20.*7.696420262413979e-21;
t72 = t3.*t15.*t20.*3.509445006623964e-21;
t74 = t8.*t15.*t20.*1.275307569480848e-20;
t75 = t4.*t15.*t20.*6.726150146755334e-23;
t76 = t8.*t15.*t20.*6.726150146755334e-23;
t77 = t15.*t20.*t29.*5.673626844500105e-17;
t79 = t7.*t15.*t20.*9.400376728708804e-20;
t82 = t3.*t15.*t20.*1.040587005840145e-22;
t28 = t27.^2;
t33 = t26.*2.228474e-2;
t34 = t25.*6.562549e-2;
t39 = t24.*3.694216783411725e-1;
t40 = t24.*1.305783216588275e-1;
t41 = t26.*1.35652563578e-4;
t43 = t26.*6.1855407534e-5;
t44 = t25.*1.656854951224248e-3;
t45 = t26.*1.834077274308e-6;
t50 = -t48;
t52 = t24.*3.215186923359161e-3;
t54 = t24.*1.345257168956303e-2;
t60 = -t58;
t61 = -t59;
t64 = t24.*1.073174736839591e-5;
t65 = t24.*4.490239736257417e-5;
t67 = t24.*3.813455334903668e-3;
t68 = t26+t47;
t78 = t15.*t20.*t30.*9.543032792050485e-17;
t81 = -t79;
t83 = -t82;
t46 = -t45;
t69 = t25+t50;
t80 = -t78;
t84 = t24.*t28.*7.997968101822611e-3;
t85 = t24.*t28.*5.407940120688672e-3;
t86 = t8.*t68.*4.334075e-2;
t87 = t24.*t28.*2.669585786930656e-5;
t88 = t24.*t28.*1.805078477303827e-5;
t89 = t24.*t28.*1.533010830938726e-3;
t90 = t24.*t28.*t29.*2.196325630278387e-1;
t91 = t24.*t28.*t30.*2.196325630278387e-1;
t93 = t4.*t68.*4.71413003675e-4;
t94 = t8.*t68.*4.71413003675e-4;
t100 = t37+t39+2.61156643317655e-1;
t101 = t38+t40+7.38843356682345e-1;
t73 = t4.*t69;
t92 = -t91;
t98 = t8.*t69.*7.0482312e-7;
t103 = t29.*t101;
t104 = t30.*t100;
t108 = t55+t77+t80;
t112 = t51+t52+t84+1.819229615328168e-2;
t115 = t32+t53+t54+t85+9.510076620873934e-3;
t95 = t73.*1.33637554986e-4;
t96 = t73.*7.26350557185e-5;
t97 = t73.*7.0482312e-7;
t99 = -t98;
t102 = t49+t73;
t105 = -t104;
t109 = t3.*t108;
t110 = t7.*t108;
t113 = t3.*t112;
t114 = t7.*t112;
t116 = t4.*t115;
t120 = t92+t103+t112;
t106 = t5.*t102.*4.36041e-5;
t107 = t9.*t102.*4.36041e-5;
t111 = -t110;
t117 = t33+t57+t114;
t118 = t34+t60+t113;
t121 = t3.*t120;
t122 = t7.*t120;
t123 = t90+t105+t115;
t119 = t8.*t117;
t124 = t4.*t123;
t126 = t33+t56+t109+t122;
t128 = t34+t61+t111+t121;
t125 = t86+t116+t119;
t127 = t8.*t126;
t129 = t86+t124+t127;
et1 = t35+t63+t65+t88-t104.*3.33783e-3+t24.*t28.*t29.*7.330961578512107e-4;
et2 = 3.174301904745164e-5;
et3 = t2.*(-6.595899203175001e-4)+t6.*2.143246017993e-3;
et4 = 4.573233567645e-4;
et5 = t6.*(t2.*2.143246017993e-3+t6.*6.595899203175001e-4+3.222314966007e-4);
et6 = -9.81e+2./1.0e+2;
et7 = t36+t62+t64+t87+t103.*3.33783e-3-t24.*t28.*t30.*7.330961578512107e-4;
et8 = 6.072279186930818e-5;
et9 = t15.*t20.*2.127584079327986e-20;
et10 = t15.*t20.*t29.*1.893760189037778e-19-t15.*t20.*t30.*3.185302114428987e-19;
et11 = t42+t44+t46+t66+t67+t81+t83+t89-t104.*2.834740764e-1-cos(q1).*4.710919801360536e-3;
et12 = sin(q1).*(-2.43593206408921e-2)+t100.*(et1+et2).*(9.81e+2./1.0e+2)-t8.*(t43+t72+t75+t93+t99+t4.*t126.*1.08769e-2-t8.*t123.*1.08769e-2).*(9.81e+2./1.0e+2)+t2.*(et3+et4).*(9.81e+2./1.0e+2);
et13 = t4.*(t41+t71+t76+t94+t97+t124.*1.08769e-2+t127.*1.08769e-2).*(9.81e+2./1.0e+2)+et5.*et6+t5.*(t70+t96+t107+t5.*t129.*7.26735e-3+t9.*t128.*7.26735e-3).*(9.81e+2./1.0e+2);
et14 = t9.*(t74+t95+t106+t5.*t128.*7.26735e-3-t9.*t129.*7.26735e-3).*(-9.81e+2./1.0e+2)+t24.*t28.*(et7+et8).*2.154595443303097;
et15 = t15.*t20.*(et9+et10).*9.361715169001526e-16+t24.*t28.*t29.*6.226013795168135e-2;
et16 = 2.695860186595471e-3;
et17 = t24.*t28.*(t36+t62+t64+t87+6.072279186930818e-5);
et18 = 2.154595443303097;
et19 = t2.*4.486342129859745e-3-t6.*3.161090981652867e-3+t42+t44+t46+t66+t67+t81+t83+t89;
et20 = t100.*(t35+t63+t65+t88+3.174301904745164e-5).*(9.81e+2./1.0e+2);
et21 = t8.*(t43+t72+t75+t93+t99+t4.*t117.*1.08769e-2-t8.*t115.*1.08769e-2).*(-9.81e+2./1.0e+2)+t4.*(t41+t71+t76+t94+t97+t116.*1.08769e-2+t119.*1.08769e-2).*(9.81e+2./1.0e+2);
et22 = t20.^2.*1.61592684475117e-3;
et23 = t5.*(t70+t96+t107+t9.*t118.*7.26735e-3+t5.*t125.*7.26735e-3).*(9.81e+2./1.0e+2)-t9.*(t74+t95+t106+t5.*t118.*7.26735e-3-t9.*t125.*7.26735e-3).*(9.81e+2./1.0e+2)+et17.*et18;
et24 = 2.695860186595471e-3;
et25 = t3.*5.316843277159623e-5;
et26 = t4.*(-3.601891949238275e-7);
et27 = t3.*t4.*5.427853659906482e-4;
et28 = t7.*t8.*6.058377458913066e-7;
et29 = t3.*1.166015146360021e-4;
et30 = t8.*(-3.601891949238275e-7);
et31 = t3.*t8.*5.427853659906482e-4;
et32 = t4.*t7.*(-6.058377458913066e-7);
et33 = t8.*3.711904660916042e-5;
et34 = t4.*t7.*6.243418693357491e-5;
et35 = t7.*t9.*3.626595104792852e-4+t9.*t31.*4.36041e-5;
et36 = t3.*t5.*t8.*(-3.626595104792852e-4);
et37 = t8.*6.829345118814501e-5;
et38 = t4.*t7.*1.148694938939344e-4;
et39 = t5.*t7.*3.626595104792852e-4+t5.*t31.*4.36041e-5;
et40 = t3.*t8.*t9.*3.626595104792852e-4;
et41 = t3.*1.576499422517851e-6;
et42 = t7.*1.424166206293785e-3+t8.*(et25+et26+et27+et28).*(9.81e+2./1.0e+2)-t4.*(et29+et30+et31+et32).*(9.81e+2./1.0e+2);
et43 = t15.*t20.*(-8.401517993167113e-21)+t5.*(et33+et34+et35+et36).*(9.81e+2./1.0e+2)-t9.*(et37+et38+et39+et40).*(9.81e+2./1.0e+2);
et44 = t9.*(t8.*1.33637554986e-4+t5.*t8.*4.36041e-5).*(-9.81e+2./1.0e+2);
et45 = t5.*(t8.*7.26350557185e-5+t8.*t9.*4.36041e-5).*(9.81e+2./1.0e+2);
mt1 = [et11+et12+et13+et14+et15+et16,et19+et20+et21+et22+et23+et24,et41+et42+et43,et44+et45,t4.*1.33075164870018e-3-t8.*6.0680154790854e-4];
mt2 = [t5.*7.12549896598485e-4-t9.*1.31098441441266e-3];
g = real(reshape([mt1,mt2],6,1));
